simulink model "MicrogridControl"  (R2025b)
settings: Solver=VariableStepAuto  StartTime=0.0  StopTime=8  FixedStep=Ts  RelTol=1e-3
PreLoadFcn:
  | NormalOperation;
  | MicrogridControlParam;
undefined symbols (not defined in the file): base, bessModeInitial, bessSystem, bessVoltage, breakerStatus, DiscIntNeverNeededParam, ee_sli_rtmsupport, event, gcbh, generator, gflInverter, gfmInverter, Inertia, lineInductance, lineResistance, machine, plannedIsland, pmsm, powerLimit, powerQuality, PV, PVInverter, ref, resync, solar, solarInsolationChange, systemFrequency, Ts, windController, windSystem, windTurbine
libraries: nesl_utility x234, ee_lib x174, fl_lib x143, eeGeneralControl x137, simulink x78, eeTransforms x47, slpidlib x23, nesl_utility_internal x12, eePwmGenerator x9, eeSinusoidalMeasurementV2 x9, custom_lib x7, batteryecm_lib x6
(part 17 of 25)

== system MicrogridControl/Solar/Solar Plant Integrated1/Detailed/PV Plant & Controller/Controller/MPPT ==
  Qref : Inport
  ipv (A) : Inport  Port=2
  vdc (V) : Inport  Port=3
  Vabc : Inport  Port=4
  Iabc : Inport  Port=5
  Action Port : ActionPort  ActionPortLabel=if(u1 > 0)
  Solar PV Controller : Subsystem  LoadFcn=ee_sli_rtmsupport( 'loadfcn', gcbh );  mask(Solar PV Controller (Three-Phase)){L=filterInductance, frequency=frequency, iMax=iMaxPU, zBase=Vac^2/(plantRating*1000), mVAbase=plantRating*1000, VdcBase=baseVoltageDC, sampleTime=-1, Choice=Perturb and observe (P&O), Vdc=1100, delV=3, tSettling=1e-3, Kppll=100, Kipll=2000, initialPhase=0, Kpv=PV.controllerKpv, Kiv=PV.controllerKiv, Kdv=0, Kpicd=PV.controllerKpIc, Kiicd=PV.controllerKiIc, Kdicd=0, Kpicq=PV.controllerKpIc, Kiicq=PV.controllerKiIc, Kdicq=0}
      mask prompts: L "physmod:ee:library:comments:control:eeRenewablesControl:ACFilterInductanceH_MP"; frequency "physmod:ee:library:comments:control:eeRenewablesControl:SystemFrequencyHz_MP"; iMax "physmod:ee:library:comments:control:eeRenewablesControl:InverterCurrentLimitpu_MP"; zBase "physmod:ee:library:comments:control:eeRenewablesControl:BaseImpedanceACSideOhm_MP"; mVAbase "physmod:ee:library:comments:control:eeRenewablesControl:BaseMVA_MP"; VdcBase "physmod:ee:library:comments:control:eeRenewablesControl:DCBusBaseVoltageV_MP"; sampleTime "physmod:ee:library:comments:control:eeRenewablesControl:SampleTime1ForInherited_MP"; Choice "physmod:ee:library:comments:control:eeRenewablesControl:Algorithm_MP"; Vdc "physmod:ee:library:comments:control:eeRenewablesControl:InitialVoltageForMPPTV_MP"; delV "physmod:ee:library:comments:control:eeRenewablesControl:VoltageStepOfMPPTV_MP"; tSettling "physmod:ee:library:comments:control:eeRenewablesControl:SettlingTimeOfMPPTs_MP"; Kppll "physmod:ee:library:comments:control:eeRenewablesControl:ProportionalGain_MP"; Kipll "physmod:ee:library:comments:control:eeRenewablesControl:IntegralGain_MP"; initialPhase "physmod:ee:library:comments:control:eeRenewablesControl:InitialPhaseAngle_MP"; Kpv "physmod:ee:library:comments:control:eeRenewablesControl:ProportionalGain_MP"; Kiv "physmod:ee:library:comments:control:eeRenewablesControl:IntegralGain_MP"; Kdv "physmod:ee:library:comments:control:eeRenewablesControl:DerivativeGain_MP"; Kpicd "physmod:ee:library:comments:control:eeRenewablesControl:DaxisProportionalGain_MP"; Kiicd "physmod:ee:library:comments:control:eeRenewablesControl:DaxisIntegralGain_MP"; Kdicd "physmod:ee:library:comments:control:eeRenewablesControl:DaxisDerivativeGain_MP"; Kpicq "physmod:ee:library:comments:control:eeRenewablesControl:QaxisProportionalGain_MP"; Kiicq "physmod:ee:library:comments:control:eeRenewablesControl:QaxisIntegralGain_MP"; Kdicq "physmod:ee:library:comments:control:eeRenewablesControl:QaxisDerivativeGain_MP"
      mask help: physmod:ee:library:comments:control:eeRenewablesControl:PVGridFollowingController_MD
      mask init: same as MicrogridControl/Solar/Solar Plant Integrated/Detailed/PV Plant & Controller/Controller/MPPT/Solar PV Controller
      settings: CopyFcn=ee_sli_rtmsupport( 'copyfcn', gcbh );  DeleteFcn=ee_sli_rtmsupport( 'deletefcn', gcbh );  ModelCloseFcn=ee_sli_rtmsupport( 'modelclosefcn', gcbh );  PostSaveFcn=ee_sli_rtmsupport( 'postsavefcn', gcbh );  PreCopyFcn=ee_sli_rtmsupport( 'precopyfcn', gcbh );  OpenFcn=ee_sli_rtmsupport( 'openfcn', gcbh );  CloseFcn=ee_sli_rtmsupport( 'closefcn', gcbh );  PreDeleteFcn=ee_sli_rtmsupport( 'predeletefcn', gcbh );
      mask Help: web(nesl_help(gcbh))
      mask TypeOptions sampleTime: Current_controller/SystemSampleTime | DC voltage controller & current reference/SystemSampleTime
      mask TypeOptions Choice: Variant Subsystem/LabelModeActiveChoice
      mask DialogControl Container4 Prompt: physmod:ee:library:comments:control:eeRenewablesControl:General_Tab
      mask DialogControl L Prompt: AC filter inductance (H)
      mask DialogControl frequency Prompt: System frequency (Hz)
      mask DialogControl iMax Prompt: Inverter current limit (pu)
      mask DialogControl zBase Prompt: Base impedance on AC side (Ohm)
      mask DialogControl mVAbase Prompt: Base power on AC side (V*A)
      mask DialogControl VdcBase Prompt: DC bus base voltage (V)
      mask DialogControl sampleTime Prompt: Sample time (-1 for inherited)
      mask DialogControl Container5 Prompt: physmod:ee:library:comments:control:eeRenewablesControl:MPPT_Tab
      mask DialogControl Choice Prompt: Algorithm
      mask DialogControl Vdc Prompt: Initial voltage for MPPT (V)
      mask DialogControl delV Prompt: Voltage step of MPPT (V)
      mask DialogControl tSettling Prompt: Settling time of MPPT (s)
      mask DialogControl Container6 Prompt: physmod:ee:library:comments:control:eeRenewablesControl:PLL_Tab
      mask DialogControl Kppll Prompt: Proportional gain
      mask DialogControl Kipll Prompt: Integral gain
      mask DialogControl initialPhase Prompt: Initial phase angle (deg)
      mask DialogControl Container7 Prompt: physmod:ee:library:comments:control:eeRenewablesControl:VoltageController_Tab
      mask DialogControl Kpv Prompt: Proportional gain
      mask DialogControl Kiv Prompt: Integral gain
      mask DialogControl Kdv Prompt: Derivative gain
      mask DialogControl Container8 Prompt: physmod:ee:library:comments:control:eeRenewablesControl:CurrentController_Tab
      mask DialogControl Kpicd Prompt: D-axis proportional gain
      mask DialogControl Kiicd Prompt: D-axis integral gain
      mask DialogControl Kdicd Prompt: D-axis derivative gain
      mask DialogControl Kpicq Prompt: Q-axis proportional gain
      mask DialogControl Kiicq Prompt: Q-axis integral gain
      mask DialogControl Kdicq Prompt: Q-axis derivative gain
      mask Display: ee.mask.drawPVcontroller;
  mabc : Outport
  wires:
  ipv (A)/1 -> Solar PV Controller/2(ipv (A))
  Iabc/1 -> Solar PV Controller/5(iabc (pu))
  Vabc/1 -> Solar PV Controller/4(vabc (pu))
  vdc (V)/1 -> Solar PV Controller/3(vdc (V))
  Qref/1 -> Solar PV Controller/1(Qref (pu))
  Solar PV Controller/1(vabcRef (pu)) -> mabc/1

== system MicrogridControl/Solar/Solar Plant Integrated1/Detailed/PV Plant & Controller/Controller/Power Reference ==
  Iabc : Inport
  Vabc : Inport  Port=2
  PRef : Inport  Port=3
  QRef : Inport  Port=4
  Action Port : ActionPort  ActionPortLabel=else
  Power Reference Controller : Subsystem  mask(Power Reference Controller){frequency=frequency, P=Real power, MVA=plantRating*1000, zbase=Vac^2/plantRating, L=filterInductance, Imax=iMaxPU, Td=1e-3, Kpic=1.5, Kiic=10, Kd=0, kpPLL=40, kiPLL=1000, kdPLL=0}
      mask prompts: frequency "Frequency (Hz)"; P "Priority mode"; MVA "Base Power (V*A)"; zbase "Base Impedance (Ohm)"; L "Filter Inductance (H)"; Imax "Inverter current limit (pu)"; Td "Sensor time delay (s)"; Kpic "Proportional gain"; Kiic "Integral gain"; Kd "Derevative gain"; kpPLL "Proportional gain"; kiPLL "Integral gain"; kdPLL "Derevative gain"
      mask help: This block receives active and reactive power references for the converter based on system requirements or higher-level control commands. It ensures that the converter operates according to desired power setpoints, supporting grid services such as frequency regulation, voltage support, and power dispatch
      settings: CopyFcn=set_param(gcbh,'LinkStatus','none');
      mask TypeOptions P: Real power  | Reactive power
      mask DialogControl Container4 Prompt: General
      mask DialogControl Container5 Prompt: Current Controller
      mask DialogControl Container5_copy Prompt: PLL
  mabc : Outport
  wires:
  QRef/1 -> Power Reference Controller/4(Qref)
  PRef/1 -> Power Reference Controller/3(Pref)
  Power Reference Controller/1(mabc) -> mabc/1
  Vabc/1 -> Power Reference Controller/2(Vabc)
  Iabc/1 -> Power Reference Controller/1(Iabc)

== system MicrogridControl/Solar/Solar Plant Integrated1/Detailed/PV Plant & Controller/PV Plant/Converter ==
  mabc : Inport
  Average : Subsystem  VariantControl=Average
  Switching : Subsystem  VariantControl=Switching
  + : PMIOPort  Side=Left
  - : PMIOPort  Port=2  Side=Left
  ~ : PMIOPort  Port=3  Side=Right

== system MicrogridControl/Solar/Solar Plant Integrated1/Detailed/PV Plant & Controller/Sensor Dynamics/Current Measurement ==
  u : Inport
  Lead-Lag (Discrete or Continuous) : eeGeneralControl/Lead-Lag (Discrete or Continuous)  T1=0  T2=PV.controllerTSensor  B=inf  A=-inf  init_option=Inherited from block input  x0=0  Ts=Ts
  V : Outport
  wires:
  u/1 -> Lead-Lag (Discrete or Continuous)/1
  Lead-Lag (Discrete or Continuous)/1 -> V/1

== system MicrogridControl/Solar/Solar Plant Integrated1/Detailed/PV Plant & Controller/Sensor Dynamics/Voltage Measurement ==
  u : Inport
  Lead-Lag (Discrete or Continuous) : eeGeneralControl/Lead-Lag (Discrete or Continuous)  T1=0  T2=PV.controllerTSensor  B=inf  A=-inf  init_option=Inherited from block input  x0=0  Ts=Ts
  I : Outport
  wires:
  u/1 -> Lead-Lag (Discrete or Continuous)/1
  Lead-Lag (Discrete or Continuous)/1 -> I/1

== system MicrogridControl/Wind Farm/Wind Plant Integrated/Detailed/PLL/PLL & Measurements1/Subsystem ==
  Vabc : Inport
  Iabc : Inport  Port=2
  Demux : Demux  Outputs=3
  Demux1 : Demux  Outputs=3
  Park Transform : eeTransforms/Park Transform  AxisAlignment=Q-axis  PowerInvariant=off
  Park Transform1 : eeTransforms/Park Transform  AxisAlignment=Q-axis  PowerInvariant=off
  Scope : Scope  NumInputPorts=2
      settings: ActiveDisplayYMinimum=0.60773339487460509  ActiveDisplayYMaximum=1.0808268521241562  DataLoggingVariableName=ScopeData5
  "Sinusoidal Measurement (PLL, Three-Phase)" : eeSinusoidalMeasurementV2/Sinusoidal Measurement (PLL, Three-Phase)  InputFilter=on  InputNormalization=off  Kp_LF=100  Ki_LF=2000  F0=50  Theta0=0  Ts=Ts
  Terminator : Terminator
  Terminator1 : Terminator
  mag : Outport
  freq : Outport  Port=2
  angle : Outport  Port=3
  Vd : Outport  Port=4
  Vq : Outport  Port=5
  Id1 : Outport  Port=6
  Iq1 : Outport  Port=7
  wires:
  Demux/3 -> Terminator/1
  Vabc/1 -> Park Transform/1, "Sinusoidal Measurement (PLL, Three-Phase)"/1
  Park Transform/1 -> Demux/1
  Demux/1 -> Scope/1, Vd/1
  Demux/2 -> Scope/2, Vq/1
  "Sinusoidal Measurement (PLL, Three-Phase)"/2 -> angle/1, Park Transform1/2, Park Transform/2
  "Sinusoidal Measurement (PLL, Three-Phase)"/1 -> freq/1
  "Sinusoidal Measurement (PLL, Three-Phase)"/3 -> mag/1
  Park Transform1/1 -> Demux1/1
  Demux1/1 -> Id1/1
  Demux1/2 -> Iq1/1
  Demux1/3 -> Terminator1/1
  Iabc/1 -> Park Transform1/1

== system MicrogridControl/Wind Farm/Wind Plant Integrated/Detailed/Wind Turbine and Converters/Wind Controller/Machine Converter Control ==
  iabc_sens : Inport
  w_sens : Inport  Port=2
  a_sens : Inport  Port=3
  vdc_sens : Inport  Port=4
  Wind speed : Inport  Port=5
  LVRT : Inport  Port=6
  Constant : Constant  Value=0  SampleTime=-1
  Constant1 : Constant  Value=(2/3)
  Constant2 : Constant  Value=psim
  Constant3 : Constant  Value=0
  Constant4 : Constant  Value=2*pi*20
  Constant5 : Constant  Value=1000  VectorParams1D=off  SampleTime=-1
  Constant6 : Constant  Value=0
  Divide : Product  Inputs=*//
  Divide1 : Product  Inputs=*/
  Gain : Gain  Gain=p
  Gain1 : Gain  Gain=2
  Gain2 : Gain  Gain=-1
  Inverse Park Transform : eeTransforms/Inverse Park Transform  AxisAlignment=Q-axis  PowerInvariant=off
  Measurements : Subsystem
  Mux : Mux  Inputs=2
  Mux1 : Mux  Inputs=2
  PMSM Controller : eePmsmCurrentController/PMSM Current Controller with Pre-Control  Kp_id=Kdip_sm  Ki_id=Kdii_sm  Kaw_id=0  Kp_iq=Kqip_sm  Ki_iq=Kqii_sm  Kaw_iq=0  Ts=-1  Tsd=0.001  AxisPrio=Q-axis  ActZC=off  ActFF=on  idVect=[-1, 0, 1]  iqVect=[-2000, 0, 2000]  LdMatrix=Ld* ones(3, 3)  LqMatrix=Lq* ones(3, 3)  psimMatrix=psim * ones(3, 3)
  Park Transform : eeTransforms/Park Transform  AxisAlignment=Q-axis  PowerInvariant=off
  Power Controller : Subsystem
  Product : Product
  Scope3 : Scope  NumInputPorts=2
      settings: ActiveDisplayYMinimum=-0.53154558960654574  ActiveDisplayYMaximum=3.2068078785969831  DataLoggingVariableName=ScopeData23
  Selector : Selector  InputPortWidth=3  IndexOptions=Index vector (dialog)  Indices=[1 2]  OutputSizes=1
  Subsystem : Subsystem
  Switch : Switch  Criteria=u2 ~= 0  SaturateOnIntegerOverflow=off  InputSameDT=off
  Unit Delay : UnitDelay  SampleTime=-1  HasFrameUpgradeWarning=on
  SM converter control : Outport  VectorParamsAs1DForOutWhenUnconnected=off
  Chopper Control : Outport  Port=2
  wires:
  Measurements/3(theta) -> Inverse Park Transform/2, Park Transform/2
  w_sens/1 -> Measurements/2(w_sens), Scope3/1, Gain/1
  a_sens/1 -> Measurements/3(th_sens), Scope3/2
  Constant3/1 -> Mux1/1
  Gain/1 -> Switch/2, Switch/1
  Subsystem/1(Out1) -> Chopper Control/1
  Constant5/1 -> PMSM Controller/4
  vdc_sens/1 -> Measurements/4(Vdc_sens)
  Measurements/4(Vdc) -> Divide1/2, Subsystem/1(Vdc)
  Gain2/1 -> PMSM Controller/1
  Mux/1 -> Inverse Park Transform/1
  Inverse Park Transform/1 -> Gain1/1
  Switch/1 -> Divide/3
  Constant6/1 -> PMSM Controller/5
  Measurements/2(iabc) -> Park Transform/1
  Constant/1 -> Mux/2
  iabc_sens/1 -> Measurements/1(iabc_sens)
  Park Transform/1 -> Selector/1
  Constant1/1 -> Product/2
  Constant2/1 -> Divide/2
  Divide1/1 -> Unit Delay/1
  Power Controller/1(activePowerDemand) -> Product/1
  Mux1/1 -> Gain2/1
  PMSM Controller/1 -> Mux/1
  Gain1/1 -> Divide1/1
  Constant4/1 -> Switch/3
  Divide/1 -> Mux1/2
  LVRT/1 -> Subsystem/2(LVRT)
  Selector/1 -> PMSM Controller/2
  Wind speed/1 -> Power Controller/1(windSpeed)
  Unit Delay/1 -> SM converter control/1
  Measurements/1(we) -> PMSM Controller/3
  Product/1 -> Divide/1

== system MicrogridControl/Wind Farm/Wind Plant Integrated/Detailed/Wind Turbine and Converters/Wind Controller/Wind Grid-side Converter Controller ==
  QRef : Inport
  BusElementIn : Inport  Port=2  PortName=VIBus  Element=Vmag
  BusElementIn4 : Inport  Port=2  PortName=VIBus  Element=Vmag
  BusElementIn1 : Inport  Port=2  PortName=VIBus  Element=Iabc
  BusElementIn2 : Inport  Port=2  PortName=VIBus  Element=Vq
  BusElementIn3 : Inport  Port=2  PortName=VIBus  Element=Vd
  BusElementIn5 : Inport  Port=2  PortName=VIBus  Element=Theta
  BusElementIn6 : Inport  Port=2  PortName=VIBus  Element=Theta
  LVRT : Inport  Port=3
  Vdc : Inport  Port=4
  Constant : Constant  Value=Vdc
  Current_controller : Subsystem
  "DC Bus Chopper control " : Subsystem
  DC voltage controller & current reference : Subsystem
  Demux : Demux  Outputs=3
  Inverse Park Transform1 : eeTransforms/Inverse Park Transform  AxisAlignment=Q-axis  PowerInvariant=off
  Park Transform1 : eeTransforms/Park Transform  AxisAlignment=Q-axis  PowerInvariant=off
  Scope{,2..4} (4 alike) : Scope  NumInputPorts=2
      Scope settings: ActiveDisplayYMinimum=-1.2499999999999998  ActiveDisplayYMaximum=11.25  DataLoggingVariableName=ScopeData33
      Scope2 settings: ActiveDisplayYMinimum=-0.15018962460144517  ActiveDisplayYMaximum=1.3517066214130067  DataLoggingVariableName=ScopeData39
      Scope3 settings: ActiveDisplayYMinimum=-0.36488768363912377  ActiveDisplayYMaximum=0.059174456441070666  DataLoggingVariableName=ScopeData41
      Scope4 settings: ActiveDisplayYMinimum=-0.2231378360878864  ActiveDisplayYMaximum=1.3471524531554082  DataLoggingVariableName=ScopeData42
  Scope1 : Scope
      settings: ActiveDisplayYMinimum=-1  ActiveDisplayYMaximum=1  DataLoggingVariableName=ScopeData34
  Terminator : Terminator
  Unit Delay2 : UnitDelay  SampleTime=Ts  HasFrameUpgradeWarning=on
  FRT : Outport
  m_abc : Outport  Port=2
  wires:
  Constant/1 -> DC voltage controller & current reference/4(Wind_vdc)
  Vdc/1 -> DC voltage controller & current reference/3(Wind_Mpp_vdc)
  Demux/3 -> Terminator/1
  "DC Bus Chopper control "/1(Out1) -> FRT/1
  BusElementIn/1 -> "DC Bus Chopper control "/1(In1)
  QRef/1 -> DC voltage controller & current reference/1(Q_ref)
  LVRT/1 -> DC voltage controller & current reference/5(lvrt.iq)
  BusElementIn4/1 -> DC voltage controller & current reference/2(Vmag)
  BusElementIn5/1 -> Inverse Park Transform1/2
  BusElementIn6/1 -> Park Transform1/2
  Current_controller/1(Refrence_mdq0) -> Scope1/1, Inverse Park Transform1/1
  Unit Delay2/1 -> m_abc/1
  Inverse Park Transform1/1 -> Unit Delay2/1
  BusElementIn2/1 -> Scope4/2, Current_controller/6(Vq)
  Park Transform1/1 -> Demux/1
  Demux/1 -> Scope2/1, Current_controller/1(iWindd)
  Demux/2 -> Current_controller/2(iq), Scope3/1
  DC voltage controller & current reference/1(id_ref) -> Scope/1, Scope2/2, Current_controller/3(id-ref)
  DC voltage controller & current reference/2(iq_ref) -> Scope/2, Scope3/2, Current_controller/4(iqref)
  BusElementIn1/1 -> Park Transform1/1
  BusElementIn3/1 -> Scope4/1, Current_controller/5(Vd)

== system MicrogridControl/Wind Farm/Wind Plant Integrated/Detailed/Wind Turbine and Converters/Wind Plant/Back-to-Back Converters ==
  Chopper : Inport
  SM_ref : Inport  Port=2
  Grid_ref : Inport  Port=3
  Average : Subsystem  VariantControl=Average
  Switching : Subsystem  VariantControl=Switching
  In : PMIOPort  Side=Left
  ~ : PMIOPort  Port=2  Side=Right
  Vdc : Outport

== system MicrogridControl/Wind Farm/Wind Plant Integrated1/Detailed/PLL/PLL & Measurements1/Subsystem ==
  Vabc : Inport
  Iabc : Inport  Port=2
  Demux : Demux  Outputs=3
  Demux1 : Demux  Outputs=3
  Park Transform : eeTransforms/Park Transform  AxisAlignment=Q-axis  PowerInvariant=off
  Park Transform1 : eeTransforms/Park Transform  AxisAlignment=Q-axis  PowerInvariant=off
  Scope : Scope  NumInputPorts=2
      settings: ActiveDisplayYMinimum=0.95416  ActiveDisplayYMaximum=1.02793  DataLoggingVariableName=ScopeData5
  "Sinusoidal Measurement (PLL, Three-Phase)" : eeSinusoidalMeasurementV2/Sinusoidal Measurement (PLL, Three-Phase)  InputFilter=on  InputNormalization=off  Kp_LF=100  Ki_LF=2000  F0=50  Theta0=0  Ts=Ts
  Terminator : Terminator
  Terminator1 : Terminator
  mag : Outport
  freq : Outport  Port=2
  angle : Outport  Port=3
  Vd : Outport  Port=4
  Vq : Outport  Port=5
  Id1 : Outport  Port=6
  Iq1 : Outport  Port=7
  wires:
  Demux/3 -> Terminator/1
  Vabc/1 -> Park Transform/1, "Sinusoidal Measurement (PLL, Three-Phase)"/1
  Park Transform/1 -> Demux/1
  Demux/1 -> Scope/1, Vd/1
  Demux/2 -> Scope/2, Vq/1
  "Sinusoidal Measurement (PLL, Three-Phase)"/2 -> angle/1, Park Transform1/2, Park Transform/2
  "Sinusoidal Measurement (PLL, Three-Phase)"/1 -> freq/1
  "Sinusoidal Measurement (PLL, Three-Phase)"/3 -> mag/1
  Park Transform1/1 -> Demux1/1
  Demux1/1 -> Id1/1
  Demux1/2 -> Iq1/1
  Demux1/3 -> Terminator1/1
  Iabc/1 -> Park Transform1/1

== system MicrogridControl/Wind Farm/Wind Plant Integrated1/Detailed/Wind Turbine and Converters/Wind Controller/Machine Converter Control ==
  iabc_sens : Inport
  w_sens : Inport  Port=2
  a_sens : Inport  Port=3
  vdc_sens : Inport  Port=4
  Wind speed : Inport  Port=5
  LVRT : Inport  Port=6
  Constant : Constant  Value=0  SampleTime=-1
  Constant1 : Constant  Value=(2/3)
  Constant2 : Constant  Value=psim
  Constant3 : Constant  Value=0
  Constant4 : Constant  Value=2*pi*20
  Constant5 : Constant  Value=1000  VectorParams1D=off  SampleTime=-1
  Constant6 : Constant  Value=0
  Divide : Product  Inputs=*//
  Divide1 : Product  Inputs=*/
  Gain : Gain  Gain=p
  Gain1 : Gain  Gain=2
  Gain2 : Gain  Gain=-1
  Inverse Park Transform : eeTransforms/Inverse Park Transform  AxisAlignment=Q-axis  PowerInvariant=off
  Measurements : Subsystem
  Mux : Mux  Inputs=2
  Mux1 : Mux  Inputs=2
  PMSM Controller : eePmsmCurrentController/PMSM Current Controller with Pre-Control  Kp_id=Kdip_sm  Ki_id=Kdii_sm  Kaw_id=0  Kp_iq=Kqip_sm  Ki_iq=Kqii_sm  Kaw_iq=0  Ts=-1  Tsd=0.001  AxisPrio=Q-axis  ActZC=off  ActFF=on  idVect=[-1, 0, 1]  iqVect=[-2000, 0, 2000]  LdMatrix=Ld* ones(3, 3)  LqMatrix=Lq* ones(3, 3)  psimMatrix=psim * ones(3, 3)
  Park Transform : eeTransforms/Park Transform  AxisAlignment=Q-axis  PowerInvariant=off
  Power Controller : Subsystem
  Product : Product
  Scope3 : Scope  NumInputPorts=2
      settings: ActiveDisplayYMinimum=-0.53154558960654574  ActiveDisplayYMaximum=3.2068078785969831  DataLoggingVariableName=ScopeData23
  Selector : Selector  InputPortWidth=3  IndexOptions=Index vector (dialog)  Indices=[1 2]  OutputSizes=1
  Subsystem : Subsystem
  Switch : Switch  Criteria=u2 ~= 0  SaturateOnIntegerOverflow=off  InputSameDT=off
  Unit Delay : UnitDelay  SampleTime=-1  HasFrameUpgradeWarning=on
  SM converter control : Outport  VectorParamsAs1DForOutWhenUnconnected=off
  Chopper Control : Outport  Port=2
  wires:
  Measurements/3(theta) -> Inverse Park Transform/2, Park Transform/2
  w_sens/1 -> Measurements/2(w_sens), Scope3/1, Gain/1
  a_sens/1 -> Measurements/3(th_sens), Scope3/2
  Constant3/1 -> Mux1/1
  Gain/1 -> Switch/2, Switch/1
  Subsystem/1(Out1) -> Chopper Control/1
  Constant5/1 -> PMSM Controller/4
  vdc_sens/1 -> Measurements/4(Vdc_sens)
  Measurements/4(Vdc) -> Divide1/2, Subsystem/1(Vdc)
  Gain2/1 -> PMSM Controller/1
  Mux/1 -> Inverse Park Transform/1
  Inverse Park Transform/1 -> Gain1/1
  Switch/1 -> Divide/3
  Constant6/1 -> PMSM Controller/5
  Measurements/2(iabc) -> Park Transform/1
  Constant/1 -> Mux/2
  iabc_sens/1 -> Measurements/1(iabc_sens)
  Park Transform/1 -> Selector/1
  Constant1/1 -> Product/2
  Constant2/1 -> Divide/2
  Divide1/1 -> Unit Delay/1
  Power Controller/1(activePowerDemand) -> Product/1
  Mux1/1 -> Gain2/1
  PMSM Controller/1 -> Mux/1
  Gain1/1 -> Divide1/1
  Constant4/1 -> Switch/3
  Divide/1 -> Mux1/2
  LVRT/1 -> Subsystem/2(LVRT)
  Selector/1 -> PMSM Controller/2
  Wind speed/1 -> Power Controller/1(windSpeed)
  Unit Delay/1 -> SM converter control/1
  Measurements/1(we) -> PMSM Controller/3
  Product/1 -> Divide/1

== system MicrogridControl/Wind Farm/Wind Plant Integrated1/Detailed/Wind Turbine and Converters/Wind Controller/Wind Grid-side Converter Controller ==
  QRef : Inport
  BusElementIn : Inport  Port=2  PortName=VIBus  Element=Vmag
  BusElementIn4 : Inport  Port=2  PortName=VIBus  Element=Vmag
  BusElementIn1 : Inport  Port=2  PortName=VIBus  Element=Iabc
  BusElementIn2 : Inport  Port=2  PortName=VIBus  Element=Vq
  BusElementIn3 : Inport  Port=2  PortName=VIBus  Element=Vd
  BusElementIn5 : Inport  Port=2  PortName=VIBus  Element=Theta
  BusElementIn6 : Inport  Port=2  PortName=VIBus  Element=Theta
  LVRT : Inport  Port=3
  Vdc : Inport  Port=4
  Constant : Constant  Value=Vdc
  Current_controller : Subsystem
  "DC Bus Chopper control " : Subsystem
  DC voltage controller & current reference : Subsystem
  Demux : Demux  Outputs=3
  Inverse Park Transform1 : eeTransforms/Inverse Park Transform  AxisAlignment=Q-axis  PowerInvariant=off
  Park Transform1 : eeTransforms/Park Transform  AxisAlignment=Q-axis  PowerInvariant=off
  Terminator : Terminator
  Unit Delay2 : UnitDelay  SampleTime=Ts  HasFrameUpgradeWarning=on
  FRT : Outport
  m_abc : Outport  Port=2
  wires:
  Constant/1 -> DC voltage controller & current reference/4(Wind_vdc)
  Vdc/1 -> DC voltage controller & current reference/3(Wind_Mpp_vdc)
  Demux/3 -> Terminator/1
  "DC Bus Chopper control "/1(Out1) -> FRT/1
  BusElementIn/1 -> "DC Bus Chopper control "/1(In1)
  QRef/1 -> DC voltage controller & current reference/1(Q_ref)
  LVRT/1 -> DC voltage controller & current reference/5(lvrt.iq)
  BusElementIn4/1 -> DC voltage controller & current reference/2(Vmag)
  BusElementIn5/1 -> Inverse Park Transform1/2
  BusElementIn6/1 -> Park Transform1/2
  Current_controller/1(Refrence_mdq0) -> Inverse Park Transform1/1
  Unit Delay2/1 -> m_abc/1
  Inverse Park Transform1/1 -> Unit Delay2/1
  BusElementIn2/1 -> Current_controller/6(Vq)
  Park Transform1/1 -> Demux/1
  Demux/1 -> Current_controller/1(iWindd)
  Demux/2 -> Current_controller/2(iq)
  DC voltage controller & current reference/1(id_ref) -> Current_controller/3(id-ref)
  DC voltage controller & current reference/2(iq_ref) -> Current_controller/4(iqref)
  BusElementIn1/1 -> Park Transform1/1
  BusElementIn3/1 -> Current_controller/5(Vd)

== system MicrogridControl/Wind Farm/Wind Plant Integrated1/Detailed/Wind Turbine and Converters/Wind Plant/Back-to-Back Converters ==
  Chopper : Inport
  SM_ref : Inport  Port=2
  Grid_ref : Inport  Port=3
  Average : Subsystem  VariantControl=Average
  Switching : Subsystem  VariantControl=Switching
  In : PMIOPort  Side=Left
  ~ : PMIOPort  Port=2  Side=Right
  Vdc : Outport

== system MicrogridControl/BESS/BESS Integrated/Detailed/BESS Controller/Grid Following/Reference Current/Current limits ==
  Imax : Inport
  iqref : Inport  Port=2
  idref : Inport  Port=3
  Constant8 : Constant  Value=0
  Constant9 : Constant  Value=0
  Scope : Scope
      settings: ActiveDisplayYMinimum=-0.14399  ActiveDisplayYMaximum=1.29587  DataLoggingVariableName=ScopeData3
  Scope1 : Scope
      settings: ActiveDisplayYMinimum=-0.13655  ActiveDisplayYMaximum=1.22893  DataLoggingVariableName=ScopeData4
  Sqrt : Sqrt
  Sqrt1 : Sqrt
  Square{1..4} (4 alike) : Math  Operator=square
  Step2 : Step  Time=0.01  SampleTime=Ts
  Step3 : Step  Time=0.01  SampleTime=Ts
  Sum6 : Sum  Inputs=|+-
  Sum9 : Sum  Inputs=|+-
  Switch1 : Switch  Threshold=.01  SaturateOnIntegerOverflow=off  InputSameDT=off
  Switch2 : Switch  Threshold=.01  SaturateOnIntegerOverflow=off  InputSameDT=off
  iubq : Outport
  iubd : Outport  Port=2
  wires:
  idref/1 -> Square4/1
  Sqrt1/1 -> iubq/1, Scope1/1
  Imax/1 -> Square1/1, Square3/1
  Sqrt/1 -> iubd/1, Scope/1
  Constant9/1 -> Switch2/3
  Square4/1 -> Sum9/2
  Constant8/1 -> Switch1/3
  Square2/1 -> Sum6/2
  Sum6/1 -> Switch1/1
  Square3/1 -> Sum9/1
  iqref/1 -> Square2/1
  Switch1/1 -> Sqrt/1
  Square1/1 -> Sum6/1
  Switch2/1 -> Sqrt1/1
  Step2/1 -> Switch1/2
  Step3/1 -> Switch2/2
  Sum9/1 -> Switch2/1

== system MicrogridControl/BESS/BESS Integrated/Detailed/BESS Controller/Grid Following/Reference Current/Refernce id generation ==
  V_mag : Inport
  del f : Inport  Port=2
  ubid : Inport  Port=3
  PRef : Inport  Port=4
  Divide : Product  Inputs=/*
  Gain6 : Gain  Gain=-1
  P/Q Priority : Switch  Criteria=u2 ~= 0  SaturateOnIntegerOverflow=off  InputSameDT=off
  Priority Mode : Constant  Value=P-2
  Saturation Dynamic2 : simulink/Discontinuities/Saturation Dynamic  OutMin=[]  OutMax=[]  OutDataTypeStr=Inherit: Same as second input  OutDataType=fixdt(1, 16)  OutScaling=2^-10  DoSatur=off
  Saturation1 : Saturate  UpperLimit=Imax  LowerLimit=-Imax
  Scope : Scope
      settings: ActiveDisplayYMinimum=-1  ActiveDisplayYMaximum=1
  Scope1 : Scope
      settings: ActiveDisplayYMinimum=-0.68622  ActiveDisplayYMaximum=0.07625  DataLoggingVariableName=ScopeData2
  Sum : Sum  Inputs=|++
  droop m_p : Gain  Gain=mp/MVA
  ubid1 : InportShadow  Port=3
  id_ref : Outport
  wires:
  del f/1 -> droop m_p/1
  Divide/1 -> Saturation Dynamic2/2, Saturation1/1
  V_mag/1 -> Divide/1
  P/Q Priority/1 -> id_ref/1, Scope/1
  ubid1/1 -> Gain6/1
  Saturation1/1 -> P/Q Priority/1
  Priority Mode/1 -> P/Q Priority/2
  PRef/1 -> Sum/2
  Saturation Dynamic2/1 -> P/Q Priority/3, Scope1/1
  Gain6/1 -> Saturation Dynamic2/3
  ubid/1 -> Saturation Dynamic2/1
  Sum/1 -> Divide/2
  droop m_p/1 -> Sum/1

== system MicrogridControl/BESS/BESS Integrated/Detailed/BESS Controller/Grid Following/Reference Current/Refernce iq generation ==
  ubiq : Inport
  V_ref : Inport  Port=2
  V_mag : Inport  Port=3
  LVRT_iq : Inport  Port=4
  Q_ref : Inport  Port=5
  Divide1 : Product  Inputs=*/
  Gain : Gain  Gain=-1
  Gain1 : Gain  Gain=-1
  Gain7 : Gain  Gain=-1
  LVRT Priority : Switch  Threshold=.9  SaturateOnIntegerOverflow=off  InputSameDT=off
  P/Q Priority : Switch  Criteria=u2 ~= 0  SaturateOnIntegerOverflow=off  InputSameDT=off
  Priority Mode : Constant  Value=P-2
  Saturation Dynamic : simulink/Discontinuities/Saturation Dynamic  OutMin=[]  OutMax=[]  OutDataTypeStr=Inherit: Same as second input  OutDataType=fixdt(1, 16)  OutScaling=2^-10  DoSatur=off
  Saturation2 : Saturate  UpperLimit=1  LowerLimit=-1
  Saturation3 : Saturate  UpperLimit=Imax  LowerLimit=-Imax
  Sum : Sum  Inputs=|++
  Sum1 : Sum  Inputs=|-+
  droop m_v : Gain  Gain=mv
  ubiq1 : InportShadow
  iq_ref : Outport
  wires:
  Gain/1 -> iq_ref/1
  V_mag/1 -> Sum1/2, Divide1/2, LVRT Priority/2
  Q_ref/1 -> Sum/1
  Sum/1 -> Divide1/1
  droop m_v/1 -> Sum/2
  ubiq1/1 -> Gain7/1
  LVRT_iq/1 -> Saturation2/1
  V_ref/1 -> Sum1/1
  Gain7/1 -> Saturation Dynamic/3
  Saturation Dynamic/1 -> P/Q Priority/1
  Divide1/1 -> Saturation3/1, Saturation Dynamic/2
  Priority Mode/1 -> P/Q Priority/2
  Saturation3/1 -> P/Q Priority/3
  Saturation2/1 -> Gain1/1
  ubiq/1 -> Saturation Dynamic/1
  Gain1/1 -> LVRT Priority/3
  P/Q Priority/1 -> LVRT Priority/1
  Sum1/1 -> droop m_v/1
  LVRT Priority/1 -> Gain/1

== system MicrogridControl/BESS/BESS Integrated/Detailed/BESS Controller/Grid Forming/Current Limiting/CurrentLimitingMethod ==
  Igd : Inport
  Igq : Inport  Port=2
  currentLimitAndVirtual : Subsystem  VariantControl=both
  currentSaturation : Subsystem  VariantControl=ctSat
  virtualImpedance : Subsystem  VariantControl=virimp
  delVd : Outport
  delVq : Outport  Port=2
  Idmax : Outport  Port=3
  Iqmax : Outport  Port=4

== system MicrogridControl/BESS/BESS Integrated/Detailed/BESS Controller/Grid Forming/Grid Voltage Reactive Power Support/Modifying Active Power Reference ==
  PrefInput : Inport
  Vd : Inport  Port=2
  Igd : Inport  Port=3
  Igq : Inport  Port=4
  AND : Logic  IconShape=distinctive  AllPortsSameDT=off  OutDataTypeStr=boolean
  Abs : Abs  SaturateOnIntegerOverflow=off
  Compare To Constant : simulink/Logic and Bit Operations/Compare To Constant  relop=>=  const=0.95  OutDataTypeStr=boolean
  Computing New Active Power Ref : Subsystem
  Math Function1 : Math  Operator=hypot
  Power Sign : Signum
  Product : Product
  Relay : Relay  OnSwitchValue=40%maxVICurrentLimit*0.96  OffSwitchValue=1
  Scope : Scope
  Scope1 : Scope
  Scope2 : Scope
  Switch : Switch  Criteria=u2 > Threshold  SaturateOnIntegerOverflow=off  InputSameDT=off
  Pref : Outport
  wires:
  Compare To Constant/1 -> AND/1
  AND/1 -> Switch/2
  Relay/1 -> AND/2, Scope1/1
  Product/1 -> Pref/1
  Power Sign/1 -> Product/2
  Abs/1 -> Product/1
  Switch/1 -> Abs/1
  Igq/1 -> Math Function1/1, Computing New Active Power Ref/1(Iq)
  Igd/1 -> Math Function1/2
  PrefInput/1 -> Switch/3, Power Sign/1
  Vd/1 -> Compare To Constant/1, Computing New Active Power Ref/2(Vd)
  Math Function1/1 -> Relay/1, Scope2/1  "Is"
  Computing New Active Power Ref/1(Pref) -> Scope/1, Switch/1

== system MicrogridControl/BESS/BESS Integrated/Detailed/BESS Controller/Grid Forming/Grid Voltage Reactive Power Support/Modifying Reactive Power Reference ==
  Vgd : Inport
  Vgq : Inport  Port=2
  Qref : Inport  Port=3
  Pref : Inport  Port=4
  Changing the Power Reference : Subsystem
  Hysteresis : Subsystem
  Math Function : Math  Operator=hypot
  Merge : Merge
  Merge1 : Merge
  NOT : Logic  Operator=NOT  IconShape=distinctive  AllPortsSameDT=off  OutDataTypeStr=boolean
  Not Altering the Power Reference : Subsystem
  Scope : Scope
  PrefNew : Outport
  QrefNew : Outport  Port=2
  wires:
  [Qref] -> Changing the Power Reference/4(Qref)
  [Pref] -> Changing the Power Reference/3(Pref)
  Merge/1 -> PrefNew/1
  Merge1/1 -> QrefNew/1
  Pref/1 -> [Pref], Not Altering the Power Reference/1(Pref)
  Vgq/1 -> Math Function/2
  Changing the Power Reference/2(Qrefv) -> Merge1/1
  [Vd] -> Changing the Power Reference/2(Vd)
  Hysteresis/1(LVFlag) -> NOT/1, Changing the Power Reference/Enable, Scope/1
  Qref/1 -> [Qref], Not Altering the Power Reference/2(Qref)
  NOT/1 -> Not Altering the Power Reference/Enable
  Changing the Power Reference/1(Prefv) -> Merge/1
  Not Altering the Power Reference/1(Prefv) -> Merge/2
  [Vs] -> Changing the Power Reference/1(Vs)
  Math Function/1 -> [Vs], Hysteresis/1(Vs)
  Not Altering the Power Reference/2(Qrefv) -> Merge1/2
  Vgd/1 -> Math Function/1, [Vd]

== system MicrogridControl/BESS/BESS Integrated/Detailed/BESS Controller/Grid Forming/Measurement/Frequency Measurement ==
  Vabc : Inport
  Convert To PU : Gain  Gain=1/powerFreq
  Frequency Measurement : Subsystem  TreatAsAtomicUnit=on  SystemSampleTime=sampleTime  mask{initialFrequency=powerFreq, sampleTime=activePowerSampleTime}
      mask prompts: initialFrequency "Initial frequency in Hz"; sampleTime "Sample time in sec"
      mask DialogControl Container7 Prompt: General
  Low-Pass Filter : eeGeneralControl/Low-Pass Filter (Discrete or Continuous)  K=1  T=freqMeasTimeConst  B=inf  A=-inf  init_option=Inherited from block input  x0=0  Ts=-1
  freq : Outport
  wires:
  Vabc/1 -> Frequency Measurement/1(abc)
  Convert To PU/1 -> freq/1
  Frequency Measurement/1(Freq) -> Low-Pass Filter/1
  Low-Pass Filter/1 -> Convert To PU/1  "Freq"

== system MicrogridControl/BESS/BESS Integrated/Detailed/BESS Controller/Grid Forming/Measurement/abc2dq ==
  Igabc : Inport
  Angle : Inport  Port=2
  Vgabc : Inport  Port=3
  Supply Current to dq : Subsystem
  Supply Voltage  to dq1 : Subsystem
  Vgd : Outport
  Vgq : Outport  Port=2
  Igd : Outport  Port=3
  Igq : Outport  Port=4
  wires:
  Supply Voltage  to dq1/2(Vgq) -> Vgq/1  "Vgq"
  Supply Voltage  to dq1/1(Vgd) -> Vgd/1  "Vgd"
  Supply Current to dq/2(Igq) -> Igq/1  "Iq"
  Supply Current to dq/1(Igd) -> Igd/1  "Id"
  Igabc/1 -> Supply Current to dq/1(abc)
  Vgabc/1 -> Supply Voltage  to dq1/2(abc)
  Angle/1 -> Supply Current to dq/2(Angle), Supply Voltage  to dq1/1(Angle)

== system MicrogridControl/BESS/BESS Integrated/Detailed/BESS Controller/Grid Forming/Power Control/ActivePowerControl ==
  Pref : Inport
  Pmeas : Inport  Port=2
  fref : Inport  Port=3
  cntrlflag : Inport  Port=4
  fgrid : Inport  Port=5
  droopControl : Subsystem  VariantControl=droop
  vsmControl : Subsystem  VariantControl=vsm
  Theta : Outport
  w : Outport  Port=2

== system MicrogridControl/BESS/BESS Integrated/Detailed/BESS Controller/Grid Forming/Power Control/ReactiveControl ==
  note: Vs-delV
  CntrlFlag : Inport
  Qref : Inport  Port=2
  Qmeas : Inport  Port=3
  Vgdmeas : Inport  Port=4
  Vref : Inport  Port=5
  Constant2 : Constant  Value=0
  Saturation1 : Saturate  UpperLimit=(dcBusVoltage/2)/(sqrt(2/3)*girdLineVoltage)  LowerLimit=-(dcBusVoltage/2)/(sqrt(2/3)*girdLineVoltage)
  Scope : Scope
      settings: ActiveDisplayYMinimum=-1  ActiveDisplayYMaximum=1  DataLoggingVariableName=ScopeData20
  Voltage  Reference Selection : Subsystem
  Vmd : Outport
  Vmq : Outport  Port=2
  wires:
  Vgdmeas/1 -> Voltage  Reference Selection/5(Vgdmeas)
  Vref/1 -> Voltage  Reference Selection/4(Vref)
  Qmeas/1 -> Voltage  Reference Selection/3(Qmeas)
  Qref/1 -> Voltage  Reference Selection/2(Qref)
  CntrlFlag/1 -> Voltage  Reference Selection/1(cntrlflag)
  Saturation1/1 -> Vmd/1, Scope/1
  Constant2/1 -> Vmq/1
  Voltage  Reference Selection/1(Vd) -> Saturation1/1  "Q"

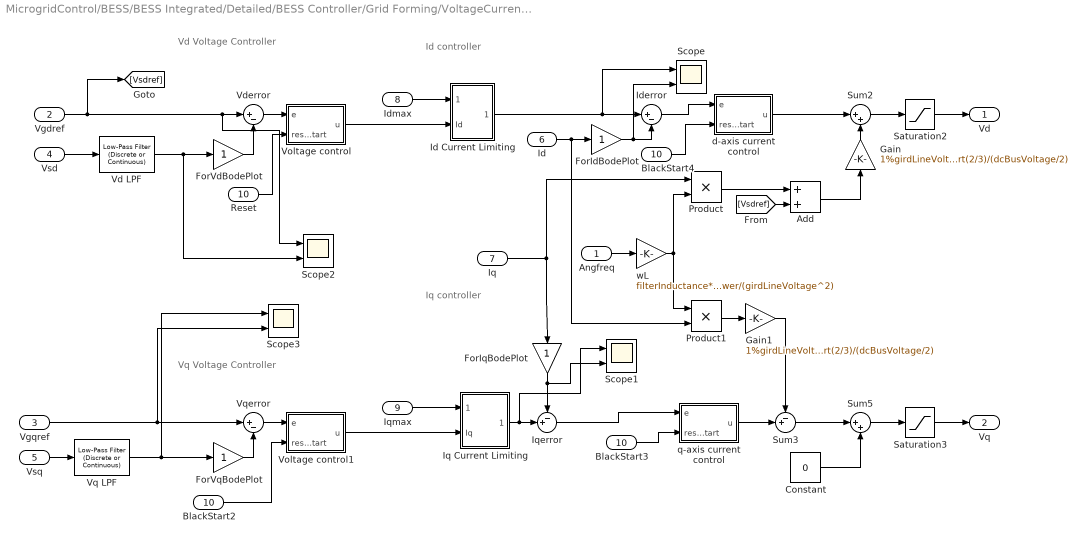
== system MicrogridControl/BESS/BESS Integrated/Detailed/BESS Controller/Grid Forming/VoltageCurrentControl/Controller ==
  note: Vq Voltage Controller
  note: Iq controller
  note: Vd Voltage Controller
  note: Id controller
  Angfreq : Inport
  Vgdref : Inport  Port=2
  Vgqref : Inport  Port=3
  Vsd : Inport  Port=4
  Vsq : Inport  Port=5
  Id : Inport  Port=6
  Iq : Inport  Port=7
  Idmax : Inport  Port=8
  Iqmax : Inport  Port=9
  Reset : Inport  Port=10
  Add : Sum
  BlackStart2 : InportShadow  Port=10
  BlackStart3 : InportShadow  Port=10
  BlackStart4 : InportShadow  Port=10
  Constant : Constant  Value=0  SampleTime=currentControlTs
  ForIdBodePlot : Gain
  ForIqBodePlot : Gain
  ForVdBodePlot : Gain
  ForVqBodePlot : Gain
  Gain : Gain  Gain=1%girdLineVoltage*sqrt(2/3)/(dcBusVoltage/2)
  Gain1 : Gain  Gain=1%girdLineVoltage*sqrt(2/3)/(dcBusVoltage/2)
  Id Current Limiting : Subsystem
  Iderror : Sum  Inputs=|+-
  Iq Current Limiting : Subsystem
  Iqerror : Sum  Inputs=-+|
  Product : Product
  Product1 : Product
  Saturation2 : Saturate  UpperLimit=4  LowerLimit=-3
  Saturation3 : Saturate  UpperLimit=3  LowerLimit=-3
  Scope{,1..3} (4 alike) : Scope  NumInputPorts=2
      Scope settings: ActiveDisplayYMinimum=-0.33488  ActiveDisplayYMaximum=2.03721
      Scope2 settings: ActiveDisplayYMinimum=-0.14129  ActiveDisplayYMaximum=1.2716
  Sum2 : Sum  Inputs=|++
  Sum3 : Sum  Inputs=-+|
  Sum5 : Sum  Inputs=|++
  Vd LPF : eeGeneralControl/Low-Pass Filter (Discrete or Continuous)  K=1  T=vdvqLPFTimeConst  B=inf  A=-inf  init_option=Specify as parameter  x0=0  Ts=voltControlTs
  Vderror : Sum  Inputs=|+-
  Voltage control : Subsystem
  Voltage control1 : Subsystem
  Vq LPF : eeGeneralControl/Low-Pass Filter (Discrete or Continuous)  K=1  T=vdvqLPFTimeConst  B=inf  A=-inf  init_option=Inherited from block input  x0=0  Ts=voltControlTs
  Vqerror : Sum  Inputs=|+-
  d-axis current control : Subsystem
  q-axis current control : Subsystem
  wL : Gain  Gain=filterInductance*power/(girdLineVoltage^2)
  Vd : Outport  VectorParamsAs1DForOutWhenUnconnected=off
  Vq : Outport  Port=2  VectorParamsAs1DForOutWhenUnconnected=off
  wires:
  Vgdref/1 -> [Vsdref], Vderror/1, Scope2/1
  BlackStart4/1 -> d-axis current control/2(resetBlackStart)
  BlackStart3/1 -> q-axis current control/2(resetBlackStart)
  BlackStart2/1 -> Voltage control1/2(resetBlackStart)
  Reset/1 -> Voltage control/2(resetBlackStart)
  Vq LPF/1 -> ForVqBodePlot/1, Scope3/1
  Vd LPF/1 -> ForVdBodePlot/1, Scope2/2
  Id Current Limiting/1(Idref) -> Iderror/1, Scope/1
  ForIqBodePlot/1 -> Iqerror/1, Scope1/2
  ForIdBodePlot/1 -> Iderror/2, Scope/2
  ForVqBodePlot/1 -> Vqerror/2
  ForVdBodePlot/1 -> Vderror/2
  Vsd/1 -> Vd LPF/1
  Voltage control1/1(u) -> Iq Current Limiting/2(Iq)
  Iq Current Limiting/1(Iqref) -> Iqerror/2, Scope1/1
  Idmax/1 -> Id Current Limiting/1(Imax)
  Voltage control/1(u) -> Id Current Limiting/2(Id)
  Gain/1 -> Sum2/2
  Add/1 -> Gain/1
  [Vsdref] -> Add/2
  Gain1/1 -> Sum3/1
  Vqerror/1 -> Voltage control1/1(e)
  Vgqref/1 -> Vqerror/1, Scope3/2
  Iqmax/1 -> Iq Current Limiting/1(Imax)
  Vderror/1 -> Voltage control/1(e)
  Id/1 -> ForIdBodePlot/1, Product1/2
  Vsq/1 -> Vq LPF/1
  Sum5/1 -> Saturation3/1
  Sum3/1 -> Sum5/1
  q-axis current control/1(u) -> Sum3/2
  Sum2/1 -> Saturation2/1
  d-axis current control/1(u) -> Sum2/1
  Product/1 -> Add/1
  Product1/1 -> Gain1/1
  Saturation2/1 -> Vd/1
  Saturation3/1 -> Vq/1
  Iderror/1 -> d-axis current control/1(e)
  Constant/1 -> Sum5/2
  Angfreq/1 -> wL/1
  Iq/1 -> Product/1, ForIqBodePlot/1
  wL/1 -> Product/2, Product1/1
  Iqerror/1 -> q-axis current control/1(e)

== system MicrogridControl/BESS/BESS Integrated/Detailed/BESS Controller/Grid Forming/VoltageCurrentControl/Modulation Signal ==
  Vd : Inport
  Vq : Inport  Port=2
  Angle : Inport  Port=3
  Constant : Constant  Value=0
  Inverse Park Transform : eeTransforms/Inverse Park Transform  AxisAlignment=D-axis  PowerInvariant=off
  Mux1 : Mux  Inputs=3
  Saturation2 : Saturate  UpperLimit=1  LowerLimit=-1
  Scope : Scope  NumInputPorts=2
      settings: DataLoggingVariableName=ScopeData9
  Scope1 : Scope
  mabc : Outport  VectorParamsAs1DForOutWhenUnconnected=off
  wires:
  Vq/1 -> Mux1/2, Scope/2
  Vd/1 -> Mux1/1, Scope/1
  Constant/1 -> Mux1/3
  Saturation2/1 -> mabc/1
  Angle/1 -> Inverse Park Transform/2, Scope1/1
  Mux1/1 -> Inverse Park Transform/1
  Inverse Park Transform/1 -> Saturation2/1

== system MicrogridControl/BESS/BESS Integrated/Detailed/BESS Plant/Converter/Switching/Pulse Generation ==
  G : Inport
  Constant : Constant  Value=5
  Subtract : Sum  Inputs=-+
  G1 : Outport  VectorParamsAs1DForOutWhenUnconnected=off
  G2 : Outport  Port=2  VectorParamsAs1DForOutWhenUnconnected=off
  wires:
  G/1 -> Subtract/1, G1/1
  Constant/1 -> Subtract/2
  Subtract/1 -> G2/1

== system MicrogridControl/BESS/BESS Integrated1/Detailed/BESS Controller/Grid Following/Reference Current/Current limits ==
  Imax : Inport
  iqref : Inport  Port=2
  idref : Inport  Port=3
  Constant8 : Constant  Value=0
  Constant9 : Constant  Value=0
  Scope : Scope
      settings: ActiveDisplayYMinimum=-0.14399  ActiveDisplayYMaximum=1.29587  DataLoggingVariableName=ScopeData3
  Scope1 : Scope
      settings: ActiveDisplayYMinimum=-0.13655  ActiveDisplayYMaximum=1.22893  DataLoggingVariableName=ScopeData4
  Sqrt : Sqrt
  Sqrt1 : Sqrt
  Square{1..4} (4 alike) : Math  Operator=square
  Step2 : Step  Time=0.01  SampleTime=Ts
  Step3 : Step  Time=0.01  SampleTime=Ts
  Sum6 : Sum  Inputs=|+-
  Sum9 : Sum  Inputs=|+-
  Switch1 : Switch  Threshold=.01  SaturateOnIntegerOverflow=off  InputSameDT=off
  Switch2 : Switch  Threshold=.01  SaturateOnIntegerOverflow=off  InputSameDT=off
  iubq : Outport
  iubd : Outport  Port=2
  wires:
  idref/1 -> Square4/1
  Sqrt1/1 -> iubq/1, Scope1/1
  Imax/1 -> Square1/1, Square3/1
  Sqrt/1 -> iubd/1, Scope/1
  Constant9/1 -> Switch2/3
  Square4/1 -> Sum9/2
  Constant8/1 -> Switch1/3
  Square2/1 -> Sum6/2
  Sum6/1 -> Switch1/1
  Square3/1 -> Sum9/1
  iqref/1 -> Square2/1
  Switch1/1 -> Sqrt/1
  Square1/1 -> Sum6/1
  Switch2/1 -> Sqrt1/1
  Step2/1 -> Switch1/2
  Step3/1 -> Switch2/2
  Sum9/1 -> Switch2/1

== system MicrogridControl/BESS/BESS Integrated1/Detailed/BESS Controller/Grid Following/Reference Current/Refernce id generation ==
  V_mag : Inport
  del f : Inport  Port=2
  ubid : Inport  Port=3
  PRef : Inport  Port=4
  Divide : Product  Inputs=/*
  Gain6 : Gain  Gain=-1
  P/Q Priority : Switch  Criteria=u2 ~= 0  SaturateOnIntegerOverflow=off  InputSameDT=off
  Priority Mode : Constant  Value=P-2
  Saturation Dynamic2 : simulink/Discontinuities/Saturation Dynamic  OutMin=[]  OutMax=[]  OutDataTypeStr=Inherit: Same as second input  OutDataType=fixdt(1, 16)  OutScaling=2^-10  DoSatur=off
  Saturation1 : Saturate  UpperLimit=Imax  LowerLimit=-Imax
  Scope : Scope
      settings: ActiveDisplayYMinimum=-1  ActiveDisplayYMaximum=1
  Scope1 : Scope
      settings: ActiveDisplayYMinimum=-0.68622  ActiveDisplayYMaximum=0.07625  DataLoggingVariableName=ScopeData2
  Sum : Sum  Inputs=|++
  droop m_p : Gain  Gain=mp/MVA
  ubid1 : InportShadow  Port=3
  id_ref : Outport
  wires:
  del f/1 -> droop m_p/1
  Divide/1 -> Saturation Dynamic2/2, Saturation1/1
  V_mag/1 -> Divide/1
  P/Q Priority/1 -> id_ref/1, Scope/1
  ubid1/1 -> Gain6/1
  Saturation1/1 -> P/Q Priority/1
  Priority Mode/1 -> P/Q Priority/2
  PRef/1 -> Sum/2
  Saturation Dynamic2/1 -> P/Q Priority/3, Scope1/1
  Gain6/1 -> Saturation Dynamic2/3
  ubid/1 -> Saturation Dynamic2/1
  Sum/1 -> Divide/2
  droop m_p/1 -> Sum/1

== system MicrogridControl/BESS/BESS Integrated1/Detailed/BESS Controller/Grid Following/Reference Current/Refernce iq generation ==
  ubiq : Inport
  V_ref : Inport  Port=2
  V_mag : Inport  Port=3
  LVRT_iq : Inport  Port=4
  Q_ref : Inport  Port=5
  Divide1 : Product  Inputs=*/
  Gain : Gain  Gain=-1
  Gain1 : Gain  Gain=-1
  Gain7 : Gain  Gain=-1
  LVRT Priority : Switch  Threshold=.9  SaturateOnIntegerOverflow=off  InputSameDT=off
  P/Q Priority : Switch  Criteria=u2 ~= 0  SaturateOnIntegerOverflow=off  InputSameDT=off
  Priority Mode : Constant  Value=P-2
  Saturation Dynamic : simulink/Discontinuities/Saturation Dynamic  OutMin=[]  OutMax=[]  OutDataTypeStr=Inherit: Same as second input  OutDataType=fixdt(1, 16)  OutScaling=2^-10  DoSatur=off
  Saturation2 : Saturate  UpperLimit=1  LowerLimit=-1
  Saturation3 : Saturate  UpperLimit=Imax  LowerLimit=-Imax
  Sum : Sum  Inputs=|++
  Sum1 : Sum  Inputs=|-+
  droop m_v : Gain  Gain=mv
  ubiq1 : InportShadow
  iq_ref : Outport
  wires:
  Gain/1 -> iq_ref/1
  V_mag/1 -> Sum1/2, Divide1/2, LVRT Priority/2
  Q_ref/1 -> Sum/1
  Sum/1 -> Divide1/1
  droop m_v/1 -> Sum/2
  ubiq1/1 -> Gain7/1
  LVRT_iq/1 -> Saturation2/1
  V_ref/1 -> Sum1/1
  Gain7/1 -> Saturation Dynamic/3
  Saturation Dynamic/1 -> P/Q Priority/1
  Divide1/1 -> Saturation3/1, Saturation Dynamic/2
  Priority Mode/1 -> P/Q Priority/2
  Saturation3/1 -> P/Q Priority/3
  Saturation2/1 -> Gain1/1
  ubiq/1 -> Saturation Dynamic/1
  Gain1/1 -> LVRT Priority/3
  P/Q Priority/1 -> LVRT Priority/1
  Sum1/1 -> droop m_v/1
  LVRT Priority/1 -> Gain/1

== system MicrogridControl/BESS/BESS Integrated1/Detailed/BESS Controller/Grid Forming/Current Limiting/CurrentLimitingMethod ==
  Igd : Inport
  Igq : Inport  Port=2
  currentLimitAndVirtual : Subsystem  VariantControl=both
  currentSaturation : Subsystem  VariantControl=ctSat
  virtualImpedance : Subsystem  VariantControl=virimp
  delVd : Outport
  delVq : Outport  Port=2
  Idmax : Outport  Port=3
  Iqmax : Outport  Port=4

== system MicrogridControl/BESS/BESS Integrated1/Detailed/BESS Controller/Grid Forming/Grid Voltage Reactive Power Support/Modifying Active Power Reference ==
  PrefInput : Inport
  Vd : Inport  Port=2
  Igd : Inport  Port=3
  Igq : Inport  Port=4
  AND : Logic  IconShape=distinctive  AllPortsSameDT=off  OutDataTypeStr=boolean
  Abs : Abs  SaturateOnIntegerOverflow=off
  Compare To Constant : simulink/Logic and Bit Operations/Compare To Constant  relop=>=  const=0.95  OutDataTypeStr=boolean
  Computing New Active Power Ref : Subsystem
  Math Function1 : Math  Operator=hypot
  Power Sign : Signum
  Product : Product
  Relay : Relay  OnSwitchValue=40%maxVICurrentLimit*0.96  OffSwitchValue=1
  Scope : Scope
  Scope1 : Scope
  Scope2 : Scope
  Switch : Switch  Criteria=u2 > Threshold  SaturateOnIntegerOverflow=off  InputSameDT=off
  Pref : Outport
  wires:
  Compare To Constant/1 -> AND/1
  AND/1 -> Switch/2
  Relay/1 -> AND/2, Scope1/1
  Product/1 -> Pref/1
  Power Sign/1 -> Product/2
  Abs/1 -> Product/1
  Switch/1 -> Abs/1
  Igq/1 -> Math Function1/1, Computing New Active Power Ref/1(Iq)
  Igd/1 -> Math Function1/2
  PrefInput/1 -> Switch/3, Power Sign/1
  Vd/1 -> Compare To Constant/1, Computing New Active Power Ref/2(Vd)
  Math Function1/1 -> Relay/1, Scope2/1  "Is"
  Computing New Active Power Ref/1(Pref) -> Scope/1, Switch/1

== system MicrogridControl/BESS/BESS Integrated1/Detailed/BESS Controller/Grid Forming/Grid Voltage Reactive Power Support/Modifying Reactive Power Reference ==
  Vgd : Inport
  Vgq : Inport  Port=2
  Qref : Inport  Port=3
  Pref : Inport  Port=4
  Changing the Power Reference : Subsystem
  Hysteresis : Subsystem
  Math Function : Math  Operator=hypot
  Merge : Merge
  Merge1 : Merge
  NOT : Logic  Operator=NOT  IconShape=distinctive  AllPortsSameDT=off  OutDataTypeStr=boolean
  Not Altering the Power Reference : Subsystem
  Scope : Scope
  PrefNew : Outport
  QrefNew : Outport  Port=2
  wires:
  [Qref] -> Changing the Power Reference/4(Qref)
  [Pref] -> Changing the Power Reference/3(Pref)
  Merge/1 -> PrefNew/1
  Merge1/1 -> QrefNew/1
  Pref/1 -> [Pref], Not Altering the Power Reference/1(Pref)
  Vgq/1 -> Math Function/2
  Changing the Power Reference/2(Qrefv) -> Merge1/1
  [Vd] -> Changing the Power Reference/2(Vd)
  Hysteresis/1(LVFlag) -> NOT/1, Changing the Power Reference/Enable, Scope/1
  Qref/1 -> [Qref], Not Altering the Power Reference/2(Qref)
  NOT/1 -> Not Altering the Power Reference/Enable
  Changing the Power Reference/1(Prefv) -> Merge/1
  Not Altering the Power Reference/1(Prefv) -> Merge/2
  [Vs] -> Changing the Power Reference/1(Vs)
  Math Function/1 -> [Vs], Hysteresis/1(Vs)
  Not Altering the Power Reference/2(Qrefv) -> Merge1/2
  Vgd/1 -> Math Function/1, [Vd]

== system MicrogridControl/BESS/BESS Integrated1/Detailed/BESS Controller/Grid Forming/Measurement/Frequency Measurement ==
  Vabc : Inport
  Convert To PU : Gain  Gain=1/powerFreq
  Frequency Measurement : Subsystem  TreatAsAtomicUnit=on  SystemSampleTime=sampleTime  mask{initialFrequency=powerFreq, sampleTime=activePowerSampleTime}
      mask prompts: initialFrequency "Initial frequency in Hz"; sampleTime "Sample time in sec"
      mask DialogControl Container7 Prompt: General
  Low-Pass Filter : eeGeneralControl/Low-Pass Filter (Discrete or Continuous)  K=1  T=freqMeasTimeConst  B=inf  A=-inf  init_option=Inherited from block input  x0=0  Ts=-1
  freq : Outport
  wires:
  Vabc/1 -> Frequency Measurement/1(abc)
  Convert To PU/1 -> freq/1
  Frequency Measurement/1(Freq) -> Low-Pass Filter/1
  Low-Pass Filter/1 -> Convert To PU/1  "Freq"

== system MicrogridControl/BESS/BESS Integrated1/Detailed/BESS Controller/Grid Forming/Measurement/abc2dq ==
  Igabc : Inport
  Angle : Inport  Port=2
  Vgabc : Inport  Port=3
  Supply Current to dq : Subsystem
  Supply Voltage  to dq1 : Subsystem
  Vgd : Outport
  Vgq : Outport  Port=2
  Igd : Outport  Port=3
  Igq : Outport  Port=4
  wires:
  Supply Voltage  to dq1/2(Vgq) -> Vgq/1  "Vgq"
  Supply Voltage  to dq1/1(Vgd) -> Vgd/1  "Vgd"
  Supply Current to dq/2(Igq) -> Igq/1  "Iq"
  Supply Current to dq/1(Igd) -> Igd/1  "Id"
  Igabc/1 -> Supply Current to dq/1(abc)
  Vgabc/1 -> Supply Voltage  to dq1/2(abc)
  Angle/1 -> Supply Current to dq/2(Angle), Supply Voltage  to dq1/1(Angle)
